simulink model "Copy_of_ActiveSupensionNonlinear"  (R2014a)
settings: Solver=ode45  StartTime=0.0  StopTime=10  RelTol=1e-3
undefined symbols (not defined in the file): b, k1, k2, k_nl, mb, mw
settings Model: Creator=MLRida  LastModifiedBy=MLRida

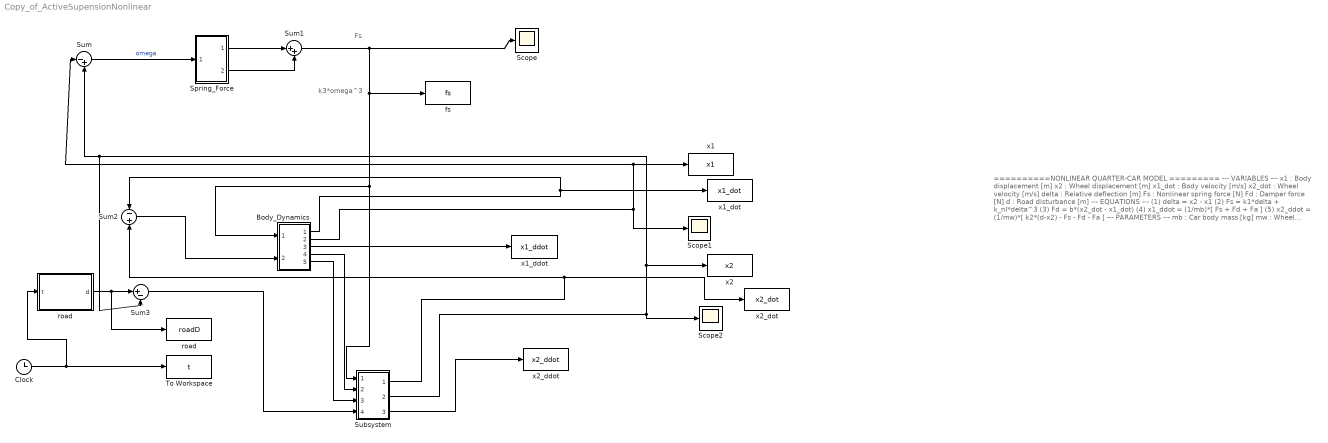
== system Copy_of_ActiveSupensionNonlinear ==
  note: Fs
  note: k3*omega^3
  note: ==========NONLINEAR QUARTER-CAR MODEL =========
      |
      | --- VARIABLES ---
      | x1 : Body displacement [m]
      | x2 : Wheel displacement [m]
      | x1_dot : Body velocity [m/s]
      | x2_dot : Wheel velocity [m/s]
      | delta : Relative deflection [m]
      | Fs : Nonlinear spring force [N]
      | Fd : Damper force [N]
      | d : Road disturbance [m]
      |
      | --- EQUATIONS ---
      | (1) delta = x2 - x1
      | (2) Fs = k1*delta + k_nl*delta^3
      | (3) Fd = b*(x2_dot - x1_dot)
      | (4) x1_ddot = (1/mb)*[ Fs + Fd + Fa ]
      | (5) x2_ddot = (1/mw)*[ k2*(d-x2) - Fs - Fd - Fa ]
      |
      | --- PARAMETERS ---
      | mb : Car body mass [kg]
      | mw : Wheel mass [kg]
      | k1 : Linear spring stiffness [N/m]
      | k_nl : Cubic nonlinear coefficient [N/m^3]
      | b : Damper coefficient [N.s/m]
      | k2 : Tyre stiffness [N/m]
      | Fa : Active actuator force [N]
      |
      | --- STATES ---
      | x = [ x1 ; x1_dot ; x2 ; x2_dot ]
      |
      | --- INPUT ---
      | u = [ Fa ; d_road ]
  Body_Dynamics : Subsystem
  Clock : Clock
  Scope : Scope
      settings: SaveName=fs
  Scope1 : Scope
      settings: SaveName=x1
  Scope2 : Scope
      settings: SaveName=x2
  Spring_Force : Subsystem
  Subsystem : Subsystem
  Sum : Sum  Inputs=|-+
  Sum1 : Sum  Inputs=|++
  Sum2 : Sum  Inputs=-|+
  Sum3 : Sum  Inputs=|+-
  To Workspace : ToWorkspace  VariableName=t  SampleTime=0.001
  fs : ToWorkspace  VariableName=fs  SampleTime=-1
  road : ToWorkspace  VariableName=roadD  SaveFormat=Structure With Time  SampleTime=0.001
  "road " : MATLAB Function  TreatAsAtomicUnit=on
  x1 : ToWorkspace  VariableName=x1  SampleTime=0.001
  x1_ddot : ToWorkspace  VariableName=x1_ddot  SampleTime=0.001
  x1_dot : ToWorkspace  VariableName=x1_dot  SampleTime=0.001
  x2 : ToWorkspace  VariableName=x2  SampleTime=0.001
  x2_ddot : ToWorkspace  VariableName=x2_ddot  SampleTime=0.001
  x2_dot : ToWorkspace  VariableName=x2_dot  SampleTime=0.001
  wires:
  Sum1/1 -> Scope/1, Subsystem/1(In1), Body_Dynamics/1(In1), fs/1
  "road "/1(d) -> road/1, Sum3/1
  Clock/1 -> "road "/1(t), To Workspace/1
  Sum/1 -> Spring_Force/1(In1)  "omega"
  Spring_Force/1(Out1) -> Sum1/1
  Spring_Force/2(Out2) -> Sum1/2
  Body_Dynamics/2(Out2) -> Scope1/1, x1/1, Sum/1
  Body_Dynamics/1(Out1) -> Sum2/1, x1_dot/1
  Sum2/1 -> Body_Dynamics/2(In2)
  Body_Dynamics/3(Out3) -> x1_ddot/1
  Subsystem/1(Out1) -> x2_dot/1, Sum2/2
  Subsystem/2(Out2) -> Scope2/1, x2/1, Sum3/2, Sum/2
  Body_Dynamics/4(Out4) -> Subsystem/2(In2)
  Body_Dynamics/5(Out5) -> Subsystem/3(In3)
  Sum3/1 -> Subsystem/4(In4)
  Subsystem/3(Out3) -> x2_ddot/1

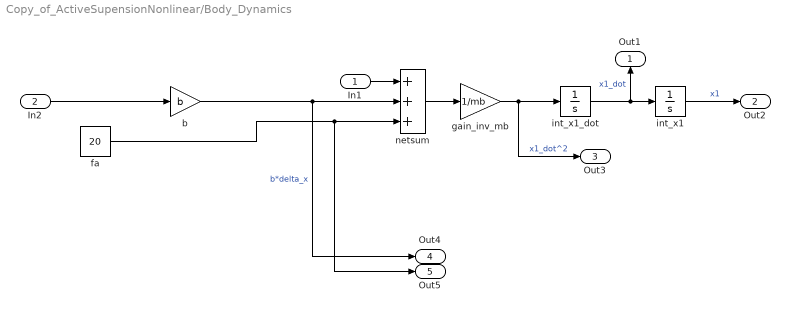
== system Copy_of_ActiveSupensionNonlinear/Body_Dynamics ==
  In1 : Inport
  In2 : Inport  Port=2
  b : Gain  Gain=b
  fa : Constant  Value=20
  gain_inv_mb : Gain  Gain=1/mb
  int_x1 : Integrator  InitialCondition=0.001
  "int_x1_dot " : Integrator  InitialCondition=0.001
  netsum : Sum  Inputs=+++  SaturateOnIntegerOverflow=on  InputSameDT=on  OutDataTypeStr=Inherit: Same as first input
  Out1 : Outport
  Out2 : Outport  Port=2
  Out3 : Outport  Port=3
  Out4 : Outport  Port=4
  Out5 : Outport  Port=5
  wires:
  gain_inv_mb/1 -> Out3/1, "int_x1_dot "/1  "x1_dot^2"
  In2/1 -> b/1
  fa/1 -> Out5/1, netsum/3
  int_x1/1 -> Out2/1  "x1"
  b/1 -> Out4/1, netsum/2  "b*delta_x"
  netsum/1 -> gain_inv_mb/1
  "int_x1_dot "/1 -> Out1/1, int_x1/1  "x1_dot"
  In1/1 -> netsum/1

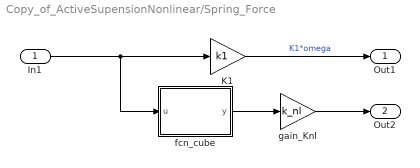
== system Copy_of_ActiveSupensionNonlinear/Spring_Force ==
  In1 : Inport
  "K1 " : Gain  Gain=k1
  "fcn_cube " : MATLAB Function  TreatAsAtomicUnit=on
  "gain_Knl " : Gain  Gain=k_nl
  Out1 : Outport
  Out2 : Outport  Port=2
  wires:
  In1/1 -> "fcn_cube "/1(u), "K1 "/1
  "gain_Knl "/1 -> Out2/1
  "K1 "/1 -> Out1/1  "K1*omega"
  "fcn_cube "/1(y) -> "gain_Knl "/1

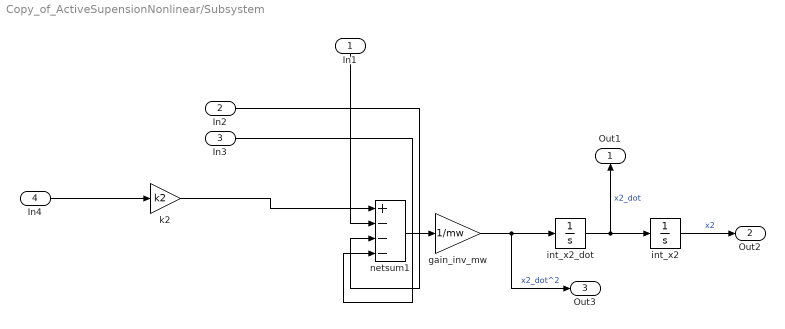
== system Copy_of_ActiveSupensionNonlinear/Subsystem ==
  In1 : Inport
  In2 : Inport  Port=2
  In3 : Inport  Port=3
  In4 : Inport  Port=4
  "gain_inv_mw " : Gain  Gain=1/mw
  int_x2 : Integrator  InitialCondition=0.001
  "int_x2_dot " : Integrator  InitialCondition=0.001
  "k2 " : Gain  Gain=k2
  netsum1 : Sum  Inputs=+---  SaturateOnIntegerOverflow=on  InputSameDT=on  OutDataTypeStr=Inherit: Same as first input
  Out1 : Outport
  Out2 : Outport  Port=2
  Out3 : Outport  Port=3
  wires:
  int_x2/1 -> Out2/1  "x2"
  "k2 "/1 -> netsum1/1
  netsum1/1 -> "gain_inv_mw "/1
  In4/1 -> "k2 "/1
  "gain_inv_mw "/1 -> Out3/1, "int_x2_dot "/1  "x2_dot^2"
  "int_x2_dot "/1 -> Out1/1, int_x2/1  "x2_dot"
  In1/1 -> netsum1/2
  In3/1 -> netsum1/4
  In2/1 -> netsum1/3

== matlab function Copy_of_ActiveSupensionNonlinear/road  ==
  data: t input; d output
function d = road_disturbance(t)
% ========================================================
%  Road Disturbance Function - Double Bump
%  --------------------------------------------------------
%  d = y1*(1 - cos(4*pi*t)),   0   <= t <= 0.5
%  d = y2*(1 - cos(4*pi*t)),   2   <= t <= 2.5
%  d = 0,                       otherwise
% ========================================================

    y1 = 0.03;    % First  bump height  [m]
    y2 = 0.05;    % Second bump height  [m]

    if t >= 0 && t <= 0.5
        d = y1 * (1 - cos(4*pi*t));

    elseif t >= 2 && t <= 2.5
        d = y2 * (1 - cos(4*pi*t));

    else
        d = 0;
    end

end

== matlab function Copy_of_ActiveSupensionNonlinear/Spring_Force/fcn_cube  ==
  data: u input; y output
function y = fcn_cube(u)
% ========================================================
%  EXTERNAL FUNCTION: Cubic Nonlinear Term
%  --------------------------------------------------------
%  Input  : u  --> delta = x2 - x1  (relative deflection)
%  Output : y  --> u^3
% ========================================================

    y = u.^3;

end
